simulink model "AcceleratorPedal"  (R2024a)
settings: Solver=VariableStepAuto  StartTime=0.0  StopTime=10.0  RelTol=1e-3
settings Model: DataDictionary=SysMLArchModel_DD.sldd  Creator=ykamatan  LastModifiedBy=ykamatan

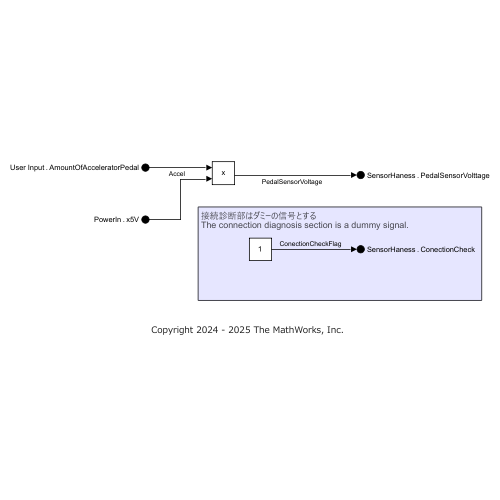
[thumbnail: Simulink's stored preview of the top-level diagram]
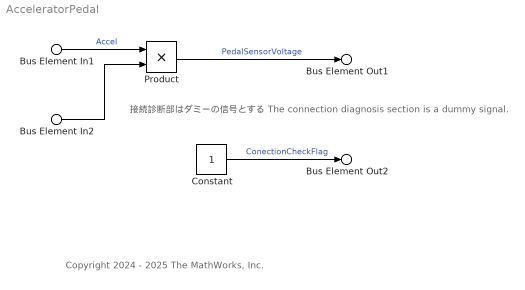
== system AcceleratorPedal ==
  note: 接続診断部はダミーの信号とする
      | The connection diagnosis section is a dummy signal.
  note: Copyright 2024 - 2025 The MathWorks, Inc.
  Bus Element In1 : Inport  PortName=User Input  Element=AmountOfAcceleratorPedal
  Bus Element In2 : Inport  Port=2  PortName=PowerIn  Element=x5V
  Constant : Constant
  Product : Product
  Bus Element Out1 : Outport  PortName=SensorHaness  Element=PedalSensorVolttage
  Bus Element Out2 : Outport  PortName=SensorHaness  Element=ConectionCheck
  wires:
  Constant/1 -> Bus Element Out2/1  "ConectionCheckFlag"
  Bus Element In1/1 -> Product/1  "Accel"
  Product/1 -> Bus Element Out1/1  "PedalSensorVoltage"
  Bus Element In2/1 -> Product/2
